simulink library "library_praktikum"  (Simulink 6.3)
libraries: dspsigops x4, dspindex x2
settings Model: LastModifiedBy=hauke  StrictBusMsg=None

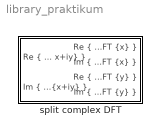
== system library_praktikum ==
  split complex DFT : Subsystem  mask(split complex DFT){size=}
      mask help:
      | This block splits the real and the imaginary part of the complex Fourier-coefficients  Z(i)=DFT{z(k)} with z(k)=x(k)+iy(k) into the real and imaginary parts of X(i)=DFT{x(k)} and Y(i)=DFT{y(k)}.
      |
      | x(k) and y(k) must be real signals.
      mask Help: Split Re{DFT{x(k)+iy(k)}} and Im{DFT{x(k)+iy(k)}} into Re{DFT{x(k)}}, Im{DFT{x(k)}, Re{DFT{y(k)}} and Im{DFT{y(k)}}.

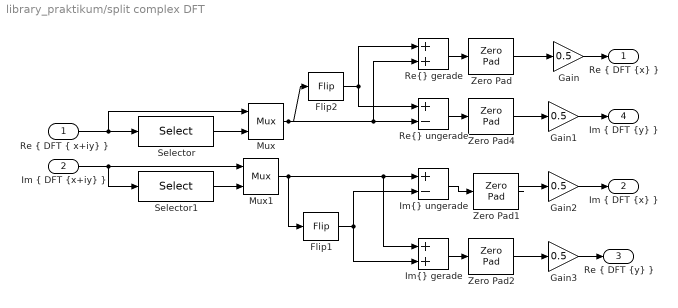
== system library_praktikum/split complex DFT ==
  "Re { DFT { x+iy} }" : Inport
  "Im { DFT {x+iy} }" : Inport  Port=2
  Flip1 : dspindex/Flip  dim=Columns
  Flip2 : dspindex/Flip  dim=Columns
  Gain{,1..3} (4 alike) : Gain  Gain=0.5  SaturateOnIntegerOverflow=on
  "Im{} gerade" : Sum  SaturateOnIntegerOverflow=on  InputSameDT=on
  "Im{} ungerade" : Sum  Inputs=+-  SaturateOnIntegerOverflow=on  InputSameDT=on
  Mux : Mux  Inputs=2
  Mux1 : Mux  Inputs=2
  "Re{} gerade" : Sum  SaturateOnIntegerOverflow=on  InputSameDT=on
  "Re{} ungerade" : Sum  Inputs=+-  SaturateOnIntegerOverflow=on  InputSameDT=on
  Selector : Selector  Elements=[1]  InputPortWidth=size
  Selector1 : Selector  Elements=[1]  InputPortWidth=size
  Zero Pad{,1..2,4} (4 alike) : dspsigops/Zero Pad  padSigAt=End  zpadAlong=Columns  padNumOutRowsSpecMethod=User-specified  numOutRows=size  padNumOutColsSpecMethod=User-specified  numOutCols=1  trunc_flag=None
  "Re { DFT {x} }" : Outport  InitialOutput=0
  "Im { DFT {x} }" : Outport  Port=2  InitialOutput=0
  "Re { DFT {y} }" : Outport  Port=3  InitialOutput=0
  "Im { DFT {y} }" : Outport  Port=4  InitialOutput=0
  wires:
  Gain3/1 -> "Re { DFT {y} }"/1
  Gain2/1 -> "Im { DFT {x} }"/1
  Gain1/1 -> "Im { DFT {y} }"/1
  Gain/1 -> "Re { DFT {x} }"/1
  Mux1/1 -> "Im{} gerade"/1, "Im{} ungerade"/1, Flip1/1
  Selector1/1 -> Mux1/2
  "Im { DFT {x+iy} }"/1 -> Selector1/1, Mux1/1
  Zero Pad2/1 -> Gain3/1
  "Im{} gerade"/1 -> Zero Pad2/1
  Zero Pad1/1 -> Gain2/1
  "Im{} ungerade"/1 -> Zero Pad1/1
  Zero Pad4/1 -> Gain1/1
  "Re{} ungerade"/1 -> Zero Pad4/1
  Zero Pad/1 -> Gain/1
  "Re{} gerade"/1 -> Zero Pad/1
  Mux/1 -> "Re{} gerade"/2, "Re{} ungerade"/2, Flip2/1
  Selector/1 -> Mux/2
  "Re { DFT { x+iy} }"/1 -> Mux/1, Selector/1
  Flip1/1 -> "Im{} gerade"/2, "Im{} ungerade"/2
  Flip2/1 -> "Re{} ungerade"/1, "Re{} gerade"/1
